simulink library "HEV_Electrical_Lib"  (R2024b)
settings: Solver=ode23t  StartTime=0.0  StopTime=10  MaxStep=1e-3  RelTol=1e-3
values from neighbouring files (symbols this model uses):
  Ts = 2e-6    (= 2e-06)    [param.m]
undefined symbols (not defined in the file or in its folder): DiscIntNeverNeededParam, HEV_Param, magnitude
libraries: fl_lib x73, nesl_utility x30, spsCurrentMeasurementLib x23, spsIdealSwitchLib x12, spsVoltageMeasurementLib x11, simulink_extras x8, spsControlledCurrentSourceLib x7, spsSeriesRLCBranchLib x6, simulink x6, spsControlledVoltageSourceLib x5, spsPermanentMagnetSynchronousMachineLib x4, spsUniversalBridgeLib x3
(part 3 of 4)

== system HEV_Electrical_Lib/Mean Value/Synchronous Motor & Drive/Torque limitation ==
  N rad/s : Inport
  Torque : Inport  Port=2
  Abs1 : Abs
  Gain : Gain  Gain=-1
  Saturation Dynamic : simulink/Discontinuities/Saturation Dynamic  OutMin=[]  OutMax=[]  OutDataTypeStr=Inherit: Same as second input  OutDataType=sfix(16)  OutScaling=2^-10  DoSatur=off
  Torque vs speed profile : Lookup  InputValues=HEV_Param.Motor.TorqSpdLUT.SpeedRPM*pi/30  Table=HEV_Param.Motor.TorqSpdLUT.TorqueNm  SaturateOnIntegerOverflow=off
  torque : Outport  VectorParamsAs1DForOutWhenUnconnected=off
  wires:
  Gain/1 -> Saturation Dynamic/3
  Torque/1 -> Saturation Dynamic/2
  Saturation Dynamic/1 -> torque/1
  Torque vs speed profile/1 -> Gain/1, Saturation Dynamic/1
  Abs1/1 -> Torque vs speed profile/1
  N rad/s/1 -> Abs1/1

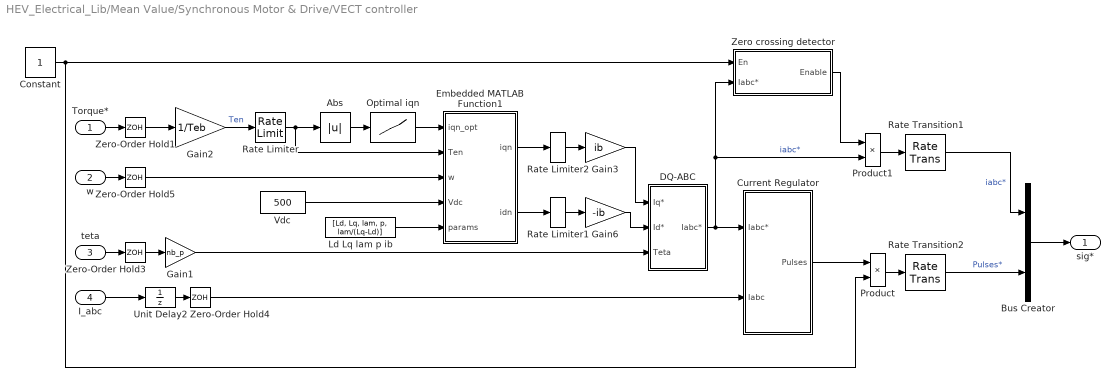
== system HEV_Electrical_Lib/Mean Value/Synchronous Motor & Drive/VECT controller ==
  Torque* : Inport
  w : Inport  Port=2
  teta : Inport  Port=3
  I_abc : Inport  Port=4
  Abs : Abs  SaturateOnIntegerOverflow=off
  Bus Creator : BusCreator  Inputs=2
  Constant : Constant
  Current Regulator : Subsystem
  DQ-ABC : Subsystem
  Embedded MATLAB Function1 : MATLAB Function  TreatAsAtomicUnit=on  SystemSampleTime=Ts_vect
  Gain1 : Gain  Gain=nb_p  SaturateOnIntegerOverflow=on  OutDataTypeStr=Inherit: Same as input  ParamDataTypeStr=Inherit: Same as input
  Gain2 : Gain  Gain=1/Teb  SaturateOnIntegerOverflow=on  OutDataTypeStr=Inherit: Same as input  ParamDataTypeStr=Inherit: Same as input
  Gain3 : Gain  Gain=ib  SaturateOnIntegerOverflow=on  OutDataTypeStr=Inherit: Same as input  ParamDataTypeStr=Inherit: Same as input
  Gain6 : Gain  Gain=-ib  SaturateOnIntegerOverflow=on  OutDataTypeStr=Inherit: Same as input  ParamDataTypeStr=Inherit: Same as input
  Ld Lq lam p ib : Constant  Value=[Ld, Lq, lam, p, lam/(Lq-Ld)]
  Optimal iqn : Lookup  InputValues=ten  Table=iqn  SaturateOnIntegerOverflow=off
  Product : Product  RndMeth=Zero
  Product1 : Product  RndMeth=Zero
  Rate Limiter : RateLimiter  RisingSlewLimit=10  FallingSlewLimit=-10  LinearizeAsGain=off
  Rate Limiter1 : RateLimiter  RisingSlewLimit=100  FallingSlewLimit=-100  SampleTimeMode=inherited
  Rate Limiter2 : RateLimiter  RisingSlewLimit=100  FallingSlewLimit=-100  SampleTimeMode=inherited
  Rate Transition1 : RateTransition
  Rate Transition2 : RateTransition
  Unit Delay2 : UnitDelay  SampleTime=-1  HasFrameUpgradeWarning=on
  Vdc : Constant  Value=500
  Zero crossing detector : Subsystem
  Zero-Order Hold{1,3..5} (4 alike) : ZeroOrderHold  SampleTime=Ts_vect
  sig* : Outport  VectorParamsAs1DForOutWhenUnconnected=off
  wires:
  Rate Limiter/1 -> Embedded MATLAB Function1/2(Ten), Abs/1
  Rate Limiter1/1 -> Gain6/1
  Rate Limiter2/1 -> Gain3/1
  Constant/1 -> Product/2, Zero crossing detector/1(En)
  Zero crossing detector/1(Enable) -> Product1/1
  Product1/1 -> Rate Transition1/1
  Product/1 -> Rate Transition2/1
  Current Regulator/1(Pulses) -> Product/1
  Rate Transition1/1 -> Bus Creator/1  "iabc*"
  Rate Transition2/1 -> Bus Creator/2  "Pulses*"
  Bus Creator/1 -> sig*/1
  Vdc/1 -> Embedded MATLAB Function1/4(Vdc)
  Abs/1 -> Optimal iqn/1
  Optimal iqn/1 -> Embedded MATLAB Function1/1(iqn_opt)
  Embedded MATLAB Function1/1(iqn) -> Rate Limiter2/1
  Ld Lq lam p ib/1 -> Embedded MATLAB Function1/5(params)
  Zero-Order Hold5/1 -> Embedded MATLAB Function1/3(w)
  Gain2/1 -> Rate Limiter/1  "Ten"
  Embedded MATLAB Function1/2(idn) -> Rate Limiter1/1
  w/1 -> Zero-Order Hold5/1
  Zero-Order Hold1/1 -> Gain2/1
  Gain6/1 -> DQ-ABC/2("Id* ")
  Gain3/1 -> DQ-ABC/1("Iq* ")
  Torque*/1 -> Zero-Order Hold1/1
  I_abc/1 -> Unit Delay2/1
  DQ-ABC/1(Iabc*) -> Product1/2, Zero crossing detector/2(Iabc*), Current Regulator/1(Iabc*)  "iabc*"
  Gain1/1 -> DQ-ABC/3(Teta)
  Zero-Order Hold3/1 -> Gain1/1
  teta/1 -> Zero-Order Hold3/1
  Zero-Order Hold4/1 -> Current Regulator/2(Iabc)
  Unit Delay2/1 -> Zero-Order Hold4/1

== system HEV_Electrical_Lib/Subsystem/System Level/Current Sensor SyncMot ==
  Current Sensor : fl_lib/Electrical/Electrical Sensors/Current Sensor
  PS-Simulink Converter : nesl_utility/PS-Simulink Converter  PhysicalDomain=network_engine_domain  SubClassName=ps_output  LeftPortType=input  RightPortType=output  PseudoPeriodic=off  Frequencies=[]  VectorFormat=1-D array  Unit=A  AffineConversion=off
  + : PMIOPort  Side=Left
  - : PMIOPort  Port=2  Side=Right
  tag scope: Mot_Current_SYS=global
  wires:
  PS-Simulink Converter/1 -> [Mot_Current_SYS]
  connections:
  -/RConn1 -- Current Sensor/RConn2
  +/RConn1 -- Current Sensor/LConn1
  Current Sensor/RConn1 -- PS-Simulink Converter/LConn1

== system HEV_Electrical_Lib/Subsystem/System Level/DC-DC Converter ==
  Calcuate Input Current Pout+PLoss = Pin : Subsystem
  Control Bus Voltage : Subsystem
  Controlled Current Source : fl_lib/Electrical/Electrical Sources/Controlled Current Source
  Controlled Voltage Source : fl_lib/Electrical/Electrical Sources/Controlled Voltage Source
  Current Sensor : Subsystem
  Load Dependant Losses : fl_lib/Electrical/Electrical Elements/Resistor  R=RLoadLoss Ohm  i_specify=off  i_priority=High  i=0 A  i_nominal_specify=off  i_nominal_value=1  i_nominal_unit=A  v_specify=off  v_priority=High  v=0 V  v_nominal_specify=off  v_nominal_value=1  v_nominal_unit=V
  PS Constant : fl_lib/Physical Signals/Sources/PS Constant  constant=Vout V
  Subsystem3 : Subsystem
      mask Display: disp('S')
  Thermal Model : Subsystem
  Voltage Sensor : Subsystem
  Voltage Sensor Bus : Subsystem
  " Batt+" : PMIOPort  Tag=PMCPort  Side=Left
  " Batt-" : PMIOPort  Tag=PMCPort  Port=2  Side=Left
  " Bus+" : PMIOPort  Tag=PMCPort  Port=3  Side=Right
  " Bus-" : PMIOPort  Tag=PMCPort  Port=4  Side=Right
  connections:
  Calcuate Input Current Pout+PLoss = Pin/RConn1 -- Subsystem3/RConn1
  Current Sensor/RConn1 -- Calcuate Input Current Pout+PLoss = Pin/LConn2
  Voltage Sensor/RConn1 -- Calcuate Input Current Pout+PLoss = Pin/LConn1
  Voltage Sensor Bus/LConn1 -- Load Dependant Losses/LConn1 -- Current Sensor/RConn2
  Current Sensor/LConn1 -- " Bus+"/RConn1
  Voltage Sensor Bus/RConn1 -- Controlled Voltage Source/RConn2 -- " Bus-"/RConn1
  Load Dependant Losses/RConn1 -- Controlled Voltage Source/LConn1
  Voltage Sensor/RConn2 -- Controlled Current Source/RConn2 -- " Batt-"/RConn1
  Voltage Sensor/LConn1 -- Controlled Current Source/LConn1 -- " Batt+"/RConn1
  Control Bus Voltage/RConn1 -- Controlled Voltage Source/RConn1
  PS Constant/RConn1 -- Control Bus Voltage/LConn2
  Subsystem3/LConn1 -- Controlled Current Source/RConn1
  Voltage Sensor Bus/RConn2 -- Control Bus Voltage/LConn1 -- Calcuate Input Current Pout+PLoss = Pin/LConn3
  Thermal Model/LConn1 -- Calcuate Input Current Pout+PLoss = Pin/RConn2

== system HEV_Electrical_Lib/Subsystem/System Level/Electrical Measurements ==
  Bus Selector : BusSelector  OutputSignals=Voltage (V),Current (A),SOC (%)
  Mux : Mux  Inputs=2
  Mux1 : Mux  Inputs=3
  Mux2 : Mux  Inputs=3
  Mux3 : Mux
  Mux4 : Mux  Inputs=2
  Product1 : Product  RndMeth=Zero
  Product2 : Product  RndMeth=Zero
  Product3 : Product  RndMeth=Zero
  tag scope: Electricals=global, Power=global
  wires:
  Mux4/1 -> Mux3/1
  Mux3/1 -> [Electricals]
  [DC_Bus_SYS] -> Mux4/2, Mux4/1, Mux/1, Product1/2, Product2/2
  Bus Selector/3 -> Mux3/4  "<SOC (%)>"
  [Gen_Current_SYS] -> Mux2/3, Product1/1
  Mux2/1 -> Mux3/3  "Current (Motor, Battery, Generator)"
  Mux/1 -> Mux3/2  "Voltage (DC bus, Battery)"
  Bus Selector/2 -> Mux2/2, Product3/2  "<Current (A)>"
  Bus Selector/1 -> Product3/1, Mux/2  "<Voltage (V)>"
  [Batt_Measures] -> Bus Selector/1
  Mux1/1 -> [Power]
  [Mot_Current_SYS] -> Mux2/1, Product2/1
  Product3/1 -> Mux1/3  "Battery power (W)"
  Product1/1 -> Mux1/2  "Generator power (W)"
  Product2/1 -> Mux1/1  "Motor Power (W)"

== system HEV_Electrical_Lib/Subsystem/System Level/Speed Sensor SyncMot ==
  MRRef : fl_lib/Mechanical/Rotational Elements/Mechanical Rotational Reference
  PS-Simulink Converter : nesl_utility/PS-Simulink Converter  PhysicalDomain=network_engine_domain  SubClassName=ps_output  LeftPortType=input  RightPortType=output  PseudoPeriodic=off  Frequencies=[]  VectorFormat=1-D array  Unit=rpm  AffineConversion=off
  Rotational Motion Sensor : fl_lib/Mechanical/Mechanical Sensors/Ideal Rotational Motion Sensor  reference=foundation.enum.MeasurementReference.difference  acceleration_port=false  velocity_port=true  position_port=true  wrap_angle=simscape.enum.onoff.off  offset=0 rad
  Sh : PMIOPort  Side=Left
  Sh1 : PMIOPort  Port=2  Side=Right
  tag scope: Mot_RPM_SYS=global
  wires:
  PS-Simulink Converter/1 -> [Mot_RPM_SYS]  "Mot_RPM"
  connections:
  Rotational Motion Sensor/RConn1 -- MRRef/LConn1
  Sh1/RConn1 -- Rotational Motion Sensor/LConn1 -- Sh/RConn1
  PS-Simulink Converter/LConn1 -- Rotational Motion Sensor/RConn2

== system HEV_Electrical_Lib/Subsystem/System Level/Synchronous Motor & Drive ==
  TReq : Inport
  GF : Subsystem
      mask Display: disp('GF')
  Inertia : fl_lib/Mechanical/Rotational Elements/Inertia  inertia=HEV_Param.Motor.Shaft_Inertia kg*m^2  num_ports=foundation.enum.numPorts2.one  w_specify=on  w_priority=High  w=0 rad/s  w_nominal_specify=off  w_nominal_value=1  w_nominal_unit=rad/s  t_specify=off  t_priority=High  t=0 N*m  t_nominal_specify=off  t_nominal_value=1  t_nominal_unit=N*m
  MRRef : fl_lib/Mechanical/Rotational Elements/Mechanical Rotational Reference
  Motor & Drive : sdl_lib/Engines & Motors/Motor & Drive  Commented=on  torque_max=10 N*m  power_max=5000 W  Tc=0.01 s  eff=100  w_eff=3750 rpm  T_eff=10 N*m  thermal_port=simscape.enum.thermaleffects.omit  thermal_mass=100 J/K  temperature_specify=off  temperature_priority=High  temperature=300 K  temperature_nominal_specify=off  temperature_nominal_value=1  temperature_nominal_unit=K
      settings: InternalSimscapePortConfiguration="{\"Bottom\":[],\"Left\":[{\"id\":\"Vp\",\"label\":\"+\",\"type\":\"foundation.electrical.electrical\"},{\"id\":\"Tr\",\"label\":\"Tr\",\"type\":\"input\"},{\"id\":\"R\",\"label\":\"R\",\"type\":\"foundation.mechanical.rotational.rotational\"}],\"Right\":[{\"id\":\"Vm\",\"label\":\"-\",\"type\":\"foundation.electrical.electrical\"},{\"id\":\"Omega\",\"label\":\"w\",\"type\":\"output\"},{\"id\":\"C\",\"label\":\"C\",\"type\":\"foundation.mechanical.rotational.rotational\"}],\"Top\":[]}"
  PS Terminator1 : Subsystem
      mask Display:
      | plot([0 0.9],[0.5 0.5]);
      | plot([0.5 0.9],[0.3 0.3]);
      | plot([0.5 0.9],[0.7 0.7]);
      | plot([0.9 0.9],[0.7 0.3]);
  Power Sensor : Subsystem
      mask Display: disp('S')
  Power and Torque Sensor : Subsystem
      mask Display: disp('S')
  Servomotor : ee_lib/Electromechanical/Motor & Drive (System Level)  torque_speed_param=1  overtorque_param=ee.enum.electromech.overtorque.no  T_t=HEV_Param.Motor.TorqSpdLUT.TorqueNm N*m  T_t_intermittent=[.36, .32, .28, 0] N*m  T_t_2D=[.09, .09, .09; .08, .08, .08; .07, .07, .07; 0, 0, 0] N*m  T_t_intermittent_2D=[.36, .36, .36; .32, .32, .32; .28, .28, .28; 0, 0, 0] N*m  w_t=HEV_Param.Motor.TorqSpdLUT.SpeedRPM rpm  vdc_t=[6, 12, 24] V  torque_max=0.1 N*m  power_max=30 W  torque_max_intermittent=0.4 N*m  power_max_intermittent=120 W  time_overtorque=30 s  time_recover=60 s  Tc=HEV_Param.Motor.TorqueControl_TimeConst s  EnableSwitch=simscape.enum.onoff.off  losses_param=1  eff=HEV_Param.Motor.Efficiency  w_eff=2000 rpm  T_eff=200 N*m  Piron=0 W  Pbase=0 W  w_eff_vec=[-8000 -4000 0 4000 8000] rpm  T_eff_vec=[0 0.03 0.06 0.09] N*m  v_eff_vec=[100, 250, 400] V  losses_mat=[1.49 1.67 2.21 3.10; 0.42 0.69 1.14 2.03; 0.06 0.24 0.78 1.68; 0.42 0.69 1.14 2.03; 1.49 1.67 2.21 3.10] W  efficiency_mat=[95 95 95 95; 95 95 95 95; 95 95 95 95; 95 95 95 95; 95 95 95 95]  losses_mat_3D=ones(5, 4, 3) W  efficiency_mat_3D=95 * ones(5, 4, 3)  Res=HEV_Param.Motor.Series_Resistance Ohm  J=0 kg*m^2  lam=HEV_Param.Motor.Damping N*m/(rad/s)  speed0=0 rpm  fault_condition=1  fault_threshold=0.5  faulted_specify=off  faulted_priority=None  faulted=0  faulted_nominal_specify=off  faulted_nominal_value=1  faulted_nominal_unit=1  isSwitchedOff_specify=off  isSwitchedOff_priority=None  isSwitchedOff=0  isSwitchedOff_nominal_specify=off  isSwitchedOff_nominal_value=1  isSwitchedOff_nominal_unit=1  torqueLimitContinuous_specify=off  torqueLimitContinuous_priority=None  torqueLimitContinuous=0 N*m  torqueLimitContinuous_nominal_specify=off  torqueLimitContinuous_nominal_value=1  torqueLimitContinuous_nominal_unit=N*m  alpha=3.93e-3 1/K  Tmeas=25 degC  Tmeas2=125 degC  losses_mat_T2=[1.49, 1.74, 2.49, 3.74; .42, .67, 1.42, 2.67; .06, .31, 1.06, 2.31; .42, .67, 1.42, 2.67; 1.49, 1.74, 2.49, 3.74] W  efficiency_mat_T2=[95, 95, 95, 95; 95, 95, 95, 95; 95, 95, 95, 95; 95, 95, 95, 95; 95, 95, 95, 95]  losses_mat_3D_T2=ones(5, 4, 3) W  efficiency_mat_3D_T2=95 * ones(5, 4, 3)  thermal_mass=100 J/K  initial_temperature=25 degC
  Vcc : PMIOPort  Side=Right
  Gnd : PMIOPort  Port=2  Side=Right
  Shaft : PMIOPort  Port=3  Side=Right
  wires:
  TReq/1 -> GF/1(In1)
  connections:
  Servomotor/RConn3 -- MRRef/LConn1
  Servomotor/LConn3 -- Power and Torque Sensor/LConn1
  Servomotor/LConn2 -- GF/RConn1
  Servomotor/LConn1 -- Power Sensor/RConn1
  Vcc/RConn1 -- Power Sensor/LConn1
  Gnd/RConn1 -- Servomotor/RConn1 -- Power Sensor/LConn2
  Servomotor/RConn2 -- PS Terminator1/LConn1
  Inertia/LConn1 -- Power and Torque Sensor/RConn1 -- Shaft/RConn1

== system HEV_Electrical_Lib/Subsystem/System Level/Voltage Sensor ==
  PS-Simulink Converter : nesl_utility/PS-Simulink Converter  PhysicalDomain=network_engine_domain  SubClassName=ps_output  LeftPortType=input  RightPortType=output  PseudoPeriodic=off  Frequencies=[]  VectorFormat=1-D array  Unit=V  AffineConversion=off
  Voltage Sensor : fl_lib/Electrical/Electrical Sensors/Voltage Sensor
  + : PMIOPort  Side=Left
  - : PMIOPort  Port=2  Side=Right
  tag scope: DC_Bus_SYS=global
  wires:
  PS-Simulink Converter/1 -> [DC_Bus_SYS]
  connections:
  -/RConn1 -- Voltage Sensor/RConn2
  +/RConn1 -- Voltage Sensor/LConn1
  Voltage Sensor/RConn1 -- PS-Simulink Converter/LConn1

== system HEV_Electrical_Lib/Detailed/DC//DC Converter/PWM/Sawtooth generator ==
  1\ib3 : Gain  Gain=2  SaturateOnIntegerOverflow=on  OutDataTypeStr=Inherit: Same as input  ParamDataTypeStr=Inherit: Same as input
  Constant1 : Constant  Value=20000
  Constant2 : Constant  Value=2
  Constant3 : Constant
  Discrete-Time Integrator : DiscreteIntegrator  IntegratorMethod=Integration: Trapezoidal  ExternalReset=rising  SampleTime=Ts  UpperSaturationLimit=1.5  LowerSaturationLimit=-1.5  ICPrevOutput=DiscIntNeverNeededParam  ICPrevScaledInput=DiscIntNeverNeededParam
  Relational Operator1 : RelationalOperator  InputSameDT=off
  Sum1 : Sum  Inputs=+-  InputSameDT=on  SaturateOnIntegerOverflow=on  OutDataTypeStr=Inherit: Same as first input
  Unit Delay : UnitDelay  SampleTime=Ts  HasFrameUpgradeWarning=on
  Out : Outport  VectorParamsAs1DForOutWhenUnconnected=off
  wires:
  Constant1/1 -> 1\ib3/1
  Discrete-Time Integrator/1 -> Relational Operator1/1, Sum1/1
  Constant2/1 -> Relational Operator1/2
  Relational Operator1/1 -> Unit Delay/1
  Unit Delay/1 -> Discrete-Time Integrator/2
  Sum1/1 -> Out/1
  Constant3/1 -> Sum1/2
  1\ib3/1 -> Discrete-Time Integrator/1

== system HEV_Electrical_Lib/Detailed/DC//DC Converter/PWM/Thermal Model ==
  IBus : Inport
  1/Mc : Gain  Gain=1/(HEV_Param.DCDCConv.Thermal_Mass*HEV_Param.DCDCConv.Specific_Heat)  SaturateOnIntegerOverflow=on  OutDataTypeStr=Inherit: Same as input  ParamDataTypeStr=Inherit: Same as input
  Air_Temp : Constant  Value=HEV_Param.DCDCConv.Air_Temperature-273
  Heat Losses : Gain  Gain=HEV_Param.DCDCConv.Convection.Area/HEV_Param.DCDCConv.Convection.HT_Coefficient  SaturateOnIntegerOverflow=on  OutDataTypeStr=Inherit: Same as input  ParamDataTypeStr=Inherit: Same as input
  Integrator : Integrator  InitialCondition=HEV_Param.DCDCConv.Initial_Temperature
  Subsystem : Subsystem
  Sum1 : Sum  Inputs=|+-  InputSameDT=on  SaturateOnIntegerOverflow=on  OutDataTypeStr=Inherit: Same as first input
  Sum2 : Sum  Inputs=|+-  InputSameDT=on  SaturateOnIntegerOverflow=on  OutDataTypeStr=Inherit: Same as first input
  tag scope: DCDC_SYS=global
  wires:
  Sum1/1 -> 1/Mc/1
  Sum2/1 -> Heat Losses/1
  Heat Losses/1 -> Sum1/2
  1/Mc/1 -> Integrator/1
  Integrator/1 -> [DCDC_SYS], Sum2/1  "DCDC_Temp"
  IBus/1 -> Subsystem/1(IBus)
  Subsystem/1(Heat Flow) -> Sum1/1  "Heat In"
  Air_Temp/1 -> Sum2/2

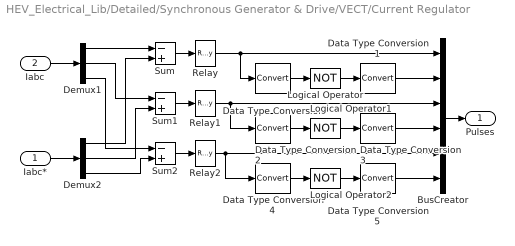
== system HEV_Electrical_Lib/Detailed/Synchronous Generator & Drive/VECT/Current Regulator ==
  Iabc* : Inport
  Iabc : Inport  Port=2
  BusCreator : BusCreator  Inputs=6
  Data Type Conversion{,1..5} (6 alike) : DataTypeConversion
  Demux1 : Demux  Outputs=3
      settings: DisplayOption=none
  Demux2 : Demux  Outputs=3
      settings: DisplayOption=none
  Logical Operator : Logic  Operator=NOT
  Logical Operator1 : Logic  Operator=NOT
  Logical Operator2 : Logic  Operator=NOT
  Relay : Relay  OnSwitchValue=h/2  OffSwitchValue=-h/2
  Relay1 : Relay  OnSwitchValue=h/2  OffSwitchValue=-h/2
  Relay2 : Relay  OnSwitchValue=h/2  OffSwitchValue=-h/2
  Sum : Sum  Inputs=-+  InputSameDT=on  SaturateOnIntegerOverflow=on  OutDataTypeStr=Inherit: Same as first input
  Sum1 : Sum  Inputs=-+  InputSameDT=on  SaturateOnIntegerOverflow=on  OutDataTypeStr=Inherit: Same as first input
  Sum2 : Sum  Inputs=-+  InputSameDT=on  SaturateOnIntegerOverflow=on  OutDataTypeStr=Inherit: Same as first input
  Pulses : Outport  InitialOutput=0  VectorParamsAs1DForOutWhenUnconnected=off
  wires:
  Logical Operator2/1 -> Data Type Conversion5/1
  Logical Operator1/1 -> Data Type Conversion3/1
  Logical Operator/1 -> Data Type Conversion1/1
  Relay2/1 -> BusCreator/5, Data Type Conversion4/1
  Relay1/1 -> BusCreator/3, Data Type Conversion2/1
  Relay/1 -> BusCreator/1, Data Type Conversion/1
  Iabc*/1 -> Demux2/1
  Demux2/1 -> Sum/2
  Demux2/2 -> Sum1/2
  Demux2/3 -> Sum2/2
  Demux1/3 -> Sum2/1
  Sum2/1 -> Relay2/1
  Iabc/1 -> Demux1/1
  BusCreator/1 -> Pulses/1
  Demux1/2 -> Sum1/1
  Demux1/1 -> Sum/1
  Sum1/1 -> Relay1/1
  Sum/1 -> Relay/1
  Data Type Conversion/1 -> Logical Operator/1
  Data Type Conversion1/1 -> BusCreator/2
  Data Type Conversion2/1 -> Logical Operator1/1
  Data Type Conversion3/1 -> BusCreator/4
  Data Type Conversion4/1 -> Logical Operator2/1
  Data Type Conversion5/1 -> BusCreator/6

== system HEV_Electrical_Lib/Detailed/Synchronous Generator & Drive/VECT/DQ-ABC ==
  "Iq* " : Inport
  "Id* " : Inport  Port=2
  Teta : Inport  Port=3
  Fcn : Fcn  Expr=sin(u)
  Fcn1 : Fcn  Expr=cos(u)
  Gain2 : Gain  SaturateOnIntegerOverflow=on  OutDataTypeStr=Inherit: Same as input  ParamDataTypeStr=Inherit: Same as input
  Gain3 : Gain  SaturateOnIntegerOverflow=on  OutDataTypeStr=Inherit: Same as input  ParamDataTypeStr=Inherit: Same as input
  Gain4 : Gain  SaturateOnIntegerOverflow=on  OutDataTypeStr=Inherit: Same as input  ParamDataTypeStr=Inherit: Same as input
  Mux : Mux
  Mux2 : Mux  Inputs=3
  ia : Fcn  Expr=-u[3]*u[2] + u[4]*u[1]
  ib : Fcn  Expr=(-u[1]+1.7320508*u[2])*u[4]*0.5+(u[2]+1.7320508*u[1])*u[3]*0.5
  ic : Sum  Inputs=--  InputSameDT=on  SaturateOnIntegerOverflow=on  OutDataTypeStr=Inherit: Same as first input
  Iabc* : Outport  InitialOutput=0  VectorParamsAs1DForOutWhenUnconnected=off
  wires:
  ib/1 -> ic/1, Gain3/1
  ia/1 -> ic/2, Gain2/1
  Gain2/1 -> Mux2/1
  Gain4/1 -> Mux2/3
  ic/1 -> Gain4/1
  Gain3/1 -> Mux2/2
  "Iq* "/1 -> Mux/4
  "Id* "/1 -> Mux/3
  Teta/1 -> Fcn/1, Fcn1/1
  Mux/1 -> ia/1, ib/1
  Mux2/1 -> Iabc*/1
  Fcn1/1 -> Mux/1
  Fcn/1 -> Mux/2

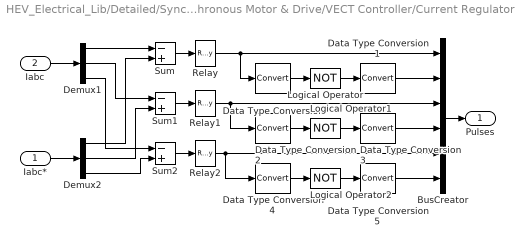
== system HEV_Electrical_Lib/Detailed/Synchronous Motor & Drive/VECT Controller/Current Regulator1 ==
  Iabc* : Inport
  Iabc : Inport  Port=2
  BusCreator : BusCreator  Inputs=6
  Data Type Conversion{,1..5} (6 alike) : DataTypeConversion
  Demux1 : Demux  Outputs=3
      settings: DisplayOption=none
  Demux2 : Demux  Outputs=3
      settings: DisplayOption=none
  Logical Operator : Logic  Operator=NOT
  Logical Operator1 : Logic  Operator=NOT
  Logical Operator2 : Logic  Operator=NOT
  Relay : Relay  OnSwitchValue=h/2  OffSwitchValue=-h/2
  Relay1 : Relay  OnSwitchValue=h/2  OffSwitchValue=-h/2
  Relay2 : Relay  OnSwitchValue=h/2  OffSwitchValue=-h/2
  Sum : Sum  Inputs=-+  InputSameDT=on  SaturateOnIntegerOverflow=on  OutDataTypeStr=Inherit: Same as first input
  Sum1 : Sum  Inputs=-+  InputSameDT=on  SaturateOnIntegerOverflow=on  OutDataTypeStr=Inherit: Same as first input
  Sum2 : Sum  Inputs=-+  InputSameDT=on  SaturateOnIntegerOverflow=on  OutDataTypeStr=Inherit: Same as first input
  Pulses : Outport  InitialOutput=0  VectorParamsAs1DForOutWhenUnconnected=off
  wires:
  Data Type Conversion5/1 -> BusCreator/6
  Data Type Conversion4/1 -> Logical Operator2/1
  Data Type Conversion3/1 -> BusCreator/4
  Data Type Conversion2/1 -> Logical Operator1/1
  Data Type Conversion1/1 -> BusCreator/2
  Data Type Conversion/1 -> Logical Operator/1
  Sum/1 -> Relay/1
  Sum1/1 -> Relay1/1
  Demux1/1 -> Sum/1
  Demux1/2 -> Sum1/1
  BusCreator/1 -> Pulses/1
  Iabc/1 -> Demux1/1
  Sum2/1 -> Relay2/1
  Demux1/3 -> Sum2/1
  Demux2/3 -> Sum2/2
  Demux2/2 -> Sum1/2
  Demux2/1 -> Sum/2
  Iabc*/1 -> Demux2/1
  Relay/1 -> Data Type Conversion/1, BusCreator/1
  Relay1/1 -> Data Type Conversion2/1, BusCreator/3
  Relay2/1 -> Data Type Conversion4/1, BusCreator/5
  Logical Operator/1 -> Data Type Conversion1/1
  Logical Operator1/1 -> Data Type Conversion3/1
  Logical Operator2/1 -> Data Type Conversion5/1

== system HEV_Electrical_Lib/Detailed/Synchronous Motor & Drive/VECT Controller/DQ-ABC ==
  "Iq* " : Inport
  "Id* " : Inport  Port=2
  Teta : Inport  Port=3
  Fcn : Fcn  Expr=sin(u)
  Fcn1 : Fcn  Expr=cos(u)
  Gain2 : Gain  SaturateOnIntegerOverflow=on  OutDataTypeStr=Inherit: Same as input  ParamDataTypeStr=Inherit: Same as input
  Gain3 : Gain  SaturateOnIntegerOverflow=on  OutDataTypeStr=Inherit: Same as input  ParamDataTypeStr=Inherit: Same as input
  Gain4 : Gain  SaturateOnIntegerOverflow=on  OutDataTypeStr=Inherit: Same as input  ParamDataTypeStr=Inherit: Same as input
  Mux : Mux
  Mux2 : Mux  Inputs=3
  ia : Fcn  Expr=-u[3]*u[2] + u[4]*u[1]
  ib : Fcn  Expr=(-u[1]+1.7320508*u[2])*u[4]*0.5+(u[2]+1.7320508*u[1])*u[3]*0.5
  ic : Sum  Inputs=--  InputSameDT=on  SaturateOnIntegerOverflow=on  OutDataTypeStr=Inherit: Same as first input
  Iabc* : Outport  InitialOutput=0  VectorParamsAs1DForOutWhenUnconnected=off
  wires:
  ib/1 -> ic/1, Gain3/1
  ia/1 -> ic/2, Gain2/1
  Gain2/1 -> Mux2/1
  Gain4/1 -> Mux2/3
  ic/1 -> Gain4/1
  Gain3/1 -> Mux2/2
  "Iq* "/1 -> Mux/4
  "Id* "/1 -> Mux/3
  Teta/1 -> Fcn/1, Fcn1/1
  Mux/1 -> ia/1, ib/1
  Mux2/1 -> Iabc*/1
  Fcn1/1 -> Mux/1
  Fcn/1 -> Mux/2

== system HEV_Electrical_Lib/Mean Value/DC//DC Converter/Boost Converter Average-Values/Thermal Model ==
  IBus : Inport
  1/Mc : Gain  Gain=1/(HEV_Param.DCDCConv.Thermal_Mass*HEV_Param.DCDCConv.Specific_Heat)  SaturateOnIntegerOverflow=on  OutDataTypeStr=Inherit: Same as input  ParamDataTypeStr=Inherit: Same as input
  Air_Temp : Constant  Value=HEV_Param.DCDCConv.Air_Temperature-273
  Heat Losses : Gain  Gain=HEV_Param.DCDCConv.Convection.Area/HEV_Param.DCDCConv.Convection.HT_Coefficient  SaturateOnIntegerOverflow=on  OutDataTypeStr=Inherit: Same as input  ParamDataTypeStr=Inherit: Same as input
  Integrator : Integrator  InitialCondition=HEV_Param.DCDCConv.Initial_Temperature
  Subsystem : Subsystem
  Sum1 : Sum  Inputs=|+-  InputSameDT=on  SaturateOnIntegerOverflow=on  OutDataTypeStr=Inherit: Same as first input
  Sum2 : Sum  Inputs=|+-  InputSameDT=on  SaturateOnIntegerOverflow=on  OutDataTypeStr=Inherit: Same as first input
  tag scope: DCDC_SYS=global
  wires:
  Air_Temp/1 -> Sum2/2
  Subsystem/1(Heat Flow) -> Sum1/1  "Heat In"
  IBus/1 -> Subsystem/1(IBus)
  Integrator/1 -> Sum2/1, [DCDC_SYS]  "DCDC_Temp"
  1/Mc/1 -> Integrator/1
  Heat Losses/1 -> Sum1/2
  Sum2/1 -> Heat Losses/1
  Sum1/1 -> 1/Mc/1

== system HEV_Electrical_Lib/Mean Value/Synchronous Generator & Drive/Three-phase Inverter/Activation Switches ==
  gate : Inport
  Ideal Switch1 : spsIdealSwitchLib/Ideal Switch  Ron=2*Ron  Lon=0  IC=1  Rs=1e6  Cs=inf  Measurements=off
  Ideal Switch2 : spsIdealSwitchLib/Ideal Switch  Ron=2*Ron  Lon=0  IC=1  Rs=1e6  Cs=inf  Measurements=off
  Ideal Switch3 : spsIdealSwitchLib/Ideal Switch  Ron=2*Ron  Lon=0  IC=1  Rs=1e6  Cs=inf  Measurements=off
  Ideal Switch4 : spsIdealSwitchLib/Ideal Switch  Ron=2*Ron  Lon=0  IC=0  Rs=1e6  Cs=inf  Measurements=off
  Ideal Switch5 : spsIdealSwitchLib/Ideal Switch  Ron=2*Ron  Lon=0  IC=0  Rs=1e6  Cs=inf  Measurements=off
  Ideal Switch6 : spsIdealSwitchLib/Ideal Switch  Ron=2*Ron  Lon=0  IC=0  Rs=1e6  Cs=inf  Measurements=off
  Logical Operator : Logic  Operator=NOT  AllPortsSameDT=off  OutDataTypeStr=boolean
  A1 : PMIOPort  Side=Left
  a : PMIOPort  Port=2  Side=Right
  B1 : PMIOPort  Port=3  Side=Left
  b : PMIOPort  Port=4  Side=Right
  C1 : PMIOPort  Port=5  Side=Left
  c : PMIOPort  Port=6  Side=Right
  A2 : PMIOPort  Port=7  Side=Left
  B2 : PMIOPort  Port=8  Side=Left
  C2 : PMIOPort  Port=9  Side=Left
  wires:
  gate/1 -> Ideal Switch1/1, Ideal Switch2/1, Ideal Switch3/1, Logical Operator/1
  Logical Operator/1 -> Ideal Switch4/1, Ideal Switch5/1, Ideal Switch6/1
  connections:
  A1/RConn1 -- Ideal Switch1/LConn1
  Ideal Switch1/RConn1 -- a/RConn1 -- Ideal Switch4/RConn1
  B1/RConn1 -- Ideal Switch2/LConn1
  Ideal Switch2/RConn1 -- Ideal Switch5/RConn1 -- b/RConn1
  C1/RConn1 -- Ideal Switch3/LConn1
  Ideal Switch3/RConn1 -- Ideal Switch6/RConn1 -- c/RConn1
  A2/RConn1 -- Ideal Switch4/LConn1
  B2/RConn1 -- Ideal Switch5/LConn1
  C2/RConn1 -- Ideal Switch6/LConn1

== system HEV_Electrical_Lib/Mean Value/Synchronous Generator & Drive/Three-phase Inverter/Id computation ==
  m : Inport
  Vdc : Inport  Port=2
  Demux : Subsystem
  Demux1 : Subsystem
  Gain : Gain  Gain=Ron
  Math Function : Math  Operator=magnitude^2  SignedPower=on
  Math Function1 : Math  Operator=magnitude^2  SignedPower=on
  Math Function2 : Math  Operator=magnitude^2  SignedPower=on
  Product1 : Product  Inputs=*/  SaturateOnIntegerOverflow=on  OutDataTypeStr=Inherit: Same as first input
  Sum1 : Sum  Inputs=+++  SaturateOnIntegerOverflow=on
  Sum2 : Sum  Inputs=|++  SaturateOnIntegerOverflow=on
  Sum3 : Sum  SaturateOnIntegerOverflow=on
  Unit Delay1 : UnitDelay  SampleTime=Ts  HasFrameUpgradeWarning=on
  Unit Delay4 : UnitDelay  InitialCondition=1  SampleTime=Ts  HasFrameUpgradeWarning=on
  Vac x Ia : Product  SaturateOnIntegerOverflow=on  OutDataTypeStr=Inherit: Same as first input
  Vbc x Ib : Product  SaturateOnIntegerOverflow=on  OutDataTypeStr=Inherit: Same as first input
  Zero avoider : Saturate  UpperLimit=inf  LowerLimit=1
  Id : Outport  VectorParamsAs1DForOutWhenUnconnected=off
  wires:
  Sum2/1 -> Unit Delay1/1
  Sum3/1 -> Sum2/1
  Sum1/1 -> Gain/1
  Math Function2/1 -> Sum1/3
  Math Function/1 -> Sum1/1
  Math Function1/1 -> Sum1/2
  Demux1/3(Ic) -> Math Function2/1
  Demux1/2(Ib) -> Math Function1/1
  Demux1/1(Ia) -> Math Function/1
  Unit Delay4/1 -> Zero avoider/1
  Unit Delay1/1 -> Product1/1
  m/1 -> Demux1/1(m), Demux/1(m)
  Vac x Ia/1 -> Sum3/1
  Vbc x Ib/1 -> Sum3/2
  Vdc/1 -> Unit Delay4/1
  Demux/1(Vac) -> Vac x Ia/1
  Demux/2(Ia) -> Vac x Ia/2
  Demux/4(Ib) -> Vbc x Ib/2
  Demux/3(Vbc) -> Vbc x Ib/1
  Gain/1 -> Sum2/2
  Product1/1 -> Id/1
  Zero avoider/1 -> Product1/2

== system HEV_Electrical_Lib/Mean Value/Synchronous Generator & Drive/Three-phase Inverter/Limit detection ==
  note: Limit = 1 saturation mode (voltage mode)
      | Limit = 0 normal mode (current mode)
  note: Low pass filter
  note: Low pass filter
  Vcc : Inport
  ctrl : Inport  Port=2
  Bus Selector1 : BusSelector  OutputSignals=m.Stator current is_d (A),m.Stator current is_q (A),m.Rotor speed wm (rad/s)  OutputAsBus=on
  Discrete Transfer Fcn1 : DiscreteTransferFcn  Numerator=[1-exp(-Ts*Fcs*2*pi)]  Denominator=[1 -exp(-Ts*Fcs*2*pi)]  SampleTime=Ts
  Discrete Transfer Fcn3 : DiscreteTransferFcn  Numerator=[1-exp(-Ts*Fcs*2*pi)]  Denominator=[1 -exp(-Ts*Fcs*2*pi)]  SampleTime=Ts
  Gain1 : Gain  Gain=0.9  SaturateOnIntegerOverflow=on  OutDataTypeStr=Inherit: Same as input  ParamDataTypeStr=Inherit: Same as input
  "Internal Vcc " : Fcn  Expr=pi/2*sqrt((Resistance*u(1)-Lq*p*u(3)*u(2))^2+(Resistance*u(2)+Ld*p*u(3)*u(1)+Flux*p*u(3))^2)
  Relational Operator : RelationalOperator  Operator=>  OutDataTypeStr=boolean  InputSameDT=off
  Relational Operator2 : RelationalOperator  Operator=<  OutDataTypeStr=boolean  InputSameDT=off
  S-R Flip-Flop : simulink_extras/Flip Flops/S-R Flip-Flop  initial_condition=0
  Terminator : Terminator
  Limit : Outport  VectorParamsAs1DForOutWhenUnconnected=off
  wires:
  Vcc/1 -> Discrete Transfer Fcn3/1
  Relational Operator/1 -> S-R Flip-Flop/1
  Relational Operator2/1 -> S-R Flip-Flop/2
  S-R Flip-Flop/1 -> Limit/1
  ctrl/1 -> Bus Selector1/1
  Bus Selector1/1 -> "Internal Vcc "/1
  "Internal Vcc "/1 -> Discrete Transfer Fcn1/1
  Discrete Transfer Fcn1/1 -> Relational Operator/1, Relational Operator2/1
  Gain1/1 -> Relational Operator2/2
  Discrete Transfer Fcn3/1 -> Gain1/1, Relational Operator/2
  S-R Flip-Flop/2 -> Terminator/1

== system HEV_Electrical_Lib/Mean Value/Synchronous Generator & Drive/Three-phase Inverter/Output Resistance correction ==
  note: Vabc
  ctrl : Inport
  1/R : Gain  Gain=1/(100*Resistance)  SaturateOnIntegerOverflow=on  OutDataTypeStr=Inherit: Same as input  ParamDataTypeStr=Inherit: Same as input
  Bus Selector1 : BusSelector  OutputSignals=m.Stator voltage Vs_d (V),m.Stator voltage Vs_q (V),m.Rotor angle thetam (rad)
  Constant : Constant  Value=0
  Discrete Transfer Fcn1 : DiscreteTransferFcn  Numerator=[1-exp(-Ts/.001)]  Denominator=[1 -exp(-Ts/.001)]  SampleTime=Ts
  Discrete Transfer Fcn2 : DiscreteTransferFcn  Numerator=[1-exp(-Ts/.001)]  Denominator=[1 -exp(-Ts/.001)]  SampleTime=Ts
  Fcn : Fcn  Expr=sin(u)
  Fcn1 : Fcn  Expr=cos(u)
  Mux4 : Mux  Inputs=3
  Mux5 : Mux  Inputs=2
  dq0_to_abc Transformation : powerlib_extras/Measurements/dq0_to_abc Transformation
  poles : Gain  Gain=p  SaturateOnIntegerOverflow=on  OutDataTypeStr=Inherit: Same as input  ParamDataTypeStr=Inherit: Same as input
  "Iabc_r " : Outport  VectorParamsAs1DForOutWhenUnconnected=off
  wires:
  1/R/1 -> "Iabc_r "/1
  Bus Selector1/2 -> Discrete Transfer Fcn2/1  "<Stator voltage Vs_q (V)>"
  Bus Selector1/1 -> Discrete Transfer Fcn1/1  "<Stator voltage Vs_d (V)>"
  ctrl/1 -> Bus Selector1/1
  Mux4/1 -> dq0_to_abc Transformation/1
  Fcn/1 -> Mux5/1
  Fcn1/1 -> Mux5/2
  Mux5/1 -> dq0_to_abc Transformation/2
  Constant/1 -> Mux4/3
  dq0_to_abc Transformation/1 -> 1/R/1
  Discrete Transfer Fcn2/1 -> Mux4/2
  Discrete Transfer Fcn1/1 -> Mux4/1
  Bus Selector1/3 -> poles/1  "<Rotor angle thetam (rad)>"
  poles/1 -> Fcn1/1, Fcn/1

== system HEV_Electrical_Lib/Mean Value/Synchronous Generator & Drive/VECT/Current Regulator ==
  Iabc* : Inport
  Iabc : Inport  Port=2
  Demux1 : Demux  Outputs=3
      settings: DisplayOption=none
  Demux2 : Demux  Outputs=3
      settings: DisplayOption=none
  Mux1 : Mux  Inputs=2
  Relay : Relay  OnSwitchValue=0  OffSwitchValue=0
  Relay1 : Relay  OnSwitchValue=0  OffSwitchValue=0
  Relay2 : Relay  OnSwitchValue=0  OffSwitchValue=0
  Sum : Sum  Inputs=-+  InputSameDT=on  SaturateOnIntegerOverflow=on  OutDataTypeStr=Inherit: Same as first input
  Sum1 : Sum  Inputs=-+  InputSameDT=on  SaturateOnIntegerOverflow=on  OutDataTypeStr=Inherit: Same as first input
  Sum2 : Sum  Inputs=-+  InputSameDT=on  SaturateOnIntegerOverflow=on  OutDataTypeStr=Inherit: Same as first input
  Sum3 : Sum  Inputs=+-
  Sum4 : Sum  Inputs=+-
  Pulses : Outport  InitialOutput=0  VectorParamsAs1DForOutWhenUnconnected=off
  wires:
  Sum/1 -> Relay/1
  Sum1/1 -> Relay1/1
  Demux1/1 -> Sum/1
  Demux1/2 -> Sum1/1
  Mux1/1 -> Pulses/1
  Iabc/1 -> Demux1/1
  Sum2/1 -> Relay2/1
  Demux1/3 -> Sum2/1
  Demux2/3 -> Sum2/2
  Demux2/2 -> Sum1/2
  Demux2/1 -> Sum/2
  Iabc*/1 -> Demux2/1
  Relay/1 -> Sum3/1
  Relay1/1 -> Sum3/2, Sum4/1
  Relay2/1 -> Sum4/2
  Sum3/1 -> Mux1/1
  Sum4/1 -> Mux1/2

== system HEV_Electrical_Lib/Mean Value/Synchronous Generator & Drive/VECT/DQ-ABC ==
  "Iq* " : Inport
  "Id* " : Inport  Port=2
  Teta : Inport  Port=3
  Fcn : Fcn  Expr=sin(u)
  Fcn1 : Fcn  Expr=cos(u)
  Gain2 : Gain  SaturateOnIntegerOverflow=on  OutDataTypeStr=Inherit: Same as input  ParamDataTypeStr=Inherit: Same as input
  Gain3 : Gain  SaturateOnIntegerOverflow=on  OutDataTypeStr=Inherit: Same as input  ParamDataTypeStr=Inherit: Same as input
  Gain4 : Gain  SaturateOnIntegerOverflow=on  OutDataTypeStr=Inherit: Same as input  ParamDataTypeStr=Inherit: Same as input
  Mux : Mux
  Mux2 : Mux  Inputs=3
  ia : Fcn  Expr=-u[3]*u[2] + u[4]*u[1]
  ib : Fcn  Expr=(-u[1]+1.7320508*u[2])*u[4]*0.5+(u[2]+1.7320508*u[1])*u[3]*0.5
  ic : Sum  Inputs=--  InputSameDT=on  SaturateOnIntegerOverflow=on  OutDataTypeStr=Inherit: Same as first input
  Iabc* : Outport  InitialOutput=0  VectorParamsAs1DForOutWhenUnconnected=off
  wires:
  ib/1 -> ic/1, Gain3/1
  ia/1 -> ic/2, Gain2/1
  Gain2/1 -> Mux2/1
  Gain4/1 -> Mux2/3
  ic/1 -> Gain4/1
  Gain3/1 -> Mux2/2
  "Iq* "/1 -> Mux/4
  "Id* "/1 -> Mux/3
  Teta/1 -> Fcn/1, Fcn1/1
  Mux/1 -> ia/1, ib/1
  Mux2/1 -> Iabc*/1
  Fcn1/1 -> Mux/1
  Fcn/1 -> Mux/2

== system HEV_Electrical_Lib/Mean Value/Synchronous Generator & Drive/VECT/Zero crossing detector ==
  Iabc* : Inport
  En : Inport  Port=2
  D Latch : simulink_extras/Flip Flops/D Latch
  D Latch1 : simulink_extras/Flip Flops/D Latch
  D Latch2 : simulink_extras/Flip Flops/D Latch
  Data Type Conversion : DataTypeConversion  SaturateOnIntegerOverflow=off  RndMeth=Floor
  Data Type Conversion2 : DataTypeConversion  SaturateOnIntegerOverflow=off  RndMeth=Floor
  Demux : Demux  Outputs=3
  Hit Crossing : HitCross
  Mux : Mux  Inputs=3
  Terminator : Terminator
  Terminator1 : Terminator
  Terminator2 : Terminator
  Enable : Outport  VectorParamsAs1DForOutWhenUnconnected=off
  wires:
  Data Type Conversion/1 -> D Latch/1, D Latch1/1, D Latch2/1
  Hit Crossing/1 -> Demux/1
  Demux/2 -> D Latch1/2
  Demux/3 -> D Latch2/2
  D Latch/1 -> Mux/1
  D Latch1/1 -> Mux/2
  D Latch2/1 -> Mux/3
  Mux/1 -> Data Type Conversion2/1
  Demux/1 -> D Latch/2
  En/1 -> Data Type Conversion/1
  Iabc*/1 -> Hit Crossing/1
  Data Type Conversion2/1 -> Enable/1
  D Latch/2 -> Terminator/1
  D Latch1/2 -> Terminator1/1
  D Latch2/2 -> Terminator2/1

== system HEV_Electrical_Lib/Mean Value/Synchronous Motor & Drive/Three-phase Inverter/Activation Switches ==
  gate : Inport
  Ideal Switch1 : spsIdealSwitchLib/Ideal Switch  Ron=2*Ron  Lon=0  IC=1  Rs=1e6  Cs=inf  Measurements=off
  Ideal Switch2 : spsIdealSwitchLib/Ideal Switch  Ron=2*Ron  Lon=0  IC=1  Rs=1e6  Cs=inf  Measurements=off
  Ideal Switch3 : spsIdealSwitchLib/Ideal Switch  Ron=2*Ron  Lon=0  IC=1  Rs=1e6  Cs=inf  Measurements=off
  Ideal Switch4 : spsIdealSwitchLib/Ideal Switch  Ron=2*Ron  Lon=0  IC=0  Rs=1e6  Cs=inf  Measurements=off
  Ideal Switch5 : spsIdealSwitchLib/Ideal Switch  Ron=2*Ron  Lon=0  IC=0  Rs=1e6  Cs=inf  Measurements=off
  Ideal Switch6 : spsIdealSwitchLib/Ideal Switch  Ron=2*Ron  Lon=0  IC=0  Rs=1e6  Cs=inf  Measurements=off
  Logical Operator : Logic  Operator=NOT  AllPortsSameDT=off  OutDataTypeStr=boolean
  A1 : PMIOPort  Side=Left
  a : PMIOPort  Port=2  Side=Right
  B1 : PMIOPort  Port=3  Side=Left
  b : PMIOPort  Port=4  Side=Right
  C1 : PMIOPort  Port=5  Side=Left
  c : PMIOPort  Port=6  Side=Right
  A2 : PMIOPort  Port=7  Side=Left
  B2 : PMIOPort  Port=8  Side=Left
  C2 : PMIOPort  Port=9  Side=Left
  wires:
  Logical Operator/1 -> Ideal Switch6/1, Ideal Switch5/1, Ideal Switch4/1
  gate/1 -> Logical Operator/1, Ideal Switch3/1, Ideal Switch2/1, Ideal Switch1/1
  connections:
  C2/RConn1 -- Ideal Switch6/LConn1
  B2/RConn1 -- Ideal Switch5/LConn1
  A2/RConn1 -- Ideal Switch4/LConn1
  c/RConn1 -- Ideal Switch6/RConn1 -- Ideal Switch3/RConn1
  C1/RConn1 -- Ideal Switch3/LConn1
  b/RConn1 -- Ideal Switch5/RConn1 -- Ideal Switch2/RConn1
  B1/RConn1 -- Ideal Switch2/LConn1
  Ideal Switch4/RConn1 -- a/RConn1 -- Ideal Switch1/RConn1
  A1/RConn1 -- Ideal Switch1/LConn1

== system HEV_Electrical_Lib/Mean Value/Synchronous Motor & Drive/Three-phase Inverter/Id computation ==
  m : Inport
  Vdc : Inport  Port=2
  Demux : Subsystem
  Demux1 : Subsystem
  Gain : Gain  Gain=Ron
  Math Function : Math  Operator=magnitude^2  SignedPower=on
  Math Function1 : Math  Operator=magnitude^2  SignedPower=on
  Math Function2 : Math  Operator=magnitude^2  SignedPower=on
  Product1 : Product  Inputs=*/  SaturateOnIntegerOverflow=on  OutDataTypeStr=Inherit: Same as first input
  Sum1 : Sum  Inputs=+++  SaturateOnIntegerOverflow=on
  Sum2 : Sum  Inputs=|++  SaturateOnIntegerOverflow=on
  Sum3 : Sum  SaturateOnIntegerOverflow=on
  Unit Delay1 : UnitDelay  SampleTime=Ts  HasFrameUpgradeWarning=on
  Unit Delay4 : UnitDelay  InitialCondition=1  SampleTime=Ts  HasFrameUpgradeWarning=on
  Vac x Ia : Product  SaturateOnIntegerOverflow=on  OutDataTypeStr=Inherit: Same as first input
  Vbc x Ib : Product  SaturateOnIntegerOverflow=on  OutDataTypeStr=Inherit: Same as first input
  Zero avoider : Saturate  UpperLimit=inf  LowerLimit=1
  Id : Outport  VectorParamsAs1DForOutWhenUnconnected=off
  wires:
  Zero avoider/1 -> Product1/2
  Product1/1 -> Id/1
  Gain/1 -> Sum2/2
  Demux/3(Vbc) -> Vbc x Ib/1
  Demux/4(Ib) -> Vbc x Ib/2
  Demux/2(Ia) -> Vac x Ia/2
  Demux/1(Vac) -> Vac x Ia/1
  Vdc/1 -> Unit Delay4/1
  Vbc x Ib/1 -> Sum3/2
  Vac x Ia/1 -> Sum3/1
  m/1 -> Demux/1(m), Demux1/1(m)
  Unit Delay1/1 -> Product1/1
  Unit Delay4/1 -> Zero avoider/1
  Demux1/1(Ia) -> Math Function/1
  Demux1/2(Ib) -> Math Function1/1
  Demux1/3(Ic) -> Math Function2/1
  Math Function1/1 -> Sum1/2
  Math Function/1 -> Sum1/1
  Math Function2/1 -> Sum1/3
  Sum1/1 -> Gain/1
  Sum3/1 -> Sum2/1
  Sum2/1 -> Unit Delay1/1

== system HEV_Electrical_Lib/Mean Value/Synchronous Motor & Drive/Three-phase Inverter/Limit detection ==
  note: Low pass filter
  note: Low pass filter
  note: Limit = 1 saturation mode (voltage mode)
      | Limit = 0 normal mode (current mode)
  Vcc : Inport
  ctrl : Inport  Port=2
  Bus Selector1 : BusSelector  OutputSignals=m.Stator current is_d (A),m.Stator current is_q (A),m.Rotor speed wm (rad/s)  OutputAsBus=on
  Discrete Transfer Fcn1 : DiscreteTransferFcn  Numerator=[1-exp(-Ts*Fcs*2*pi)]  Denominator=[1 -exp(-Ts*Fcs*2*pi)]  SampleTime=Ts
  Discrete Transfer Fcn3 : DiscreteTransferFcn  Numerator=[1-exp(-Ts*Fcs*2*pi)]  Denominator=[1 -exp(-Ts*Fcs*2*pi)]  SampleTime=Ts
  Gain1 : Gain  Gain=0.9  SaturateOnIntegerOverflow=on  OutDataTypeStr=Inherit: Same as input  ParamDataTypeStr=Inherit: Same as input
  "Internal Vcc " : Fcn  Expr=pi/2*sqrt((Resistance*u(1)-Lq*p*u(3)*u(2))^2+(Resistance*u(2)+Ld*p*u(3)*u(1)+Flux*p*u(3))^2)
  Relational Operator : RelationalOperator  Operator=>  OutDataTypeStr=boolean  InputSameDT=off
  Relational Operator2 : RelationalOperator  Operator=<  OutDataTypeStr=boolean  InputSameDT=off
  S-R Flip-Flop : simulink_extras/Flip Flops/S-R Flip-Flop  initial_condition=0
  Terminator : Terminator
  Limit : Outport  VectorParamsAs1DForOutWhenUnconnected=off
  wires:
  S-R Flip-Flop/2 -> Terminator/1
  Discrete Transfer Fcn3/1 -> Relational Operator/2, Gain1/1
  Gain1/1 -> Relational Operator2/2
  Discrete Transfer Fcn1/1 -> Relational Operator2/1, Relational Operator/1
  "Internal Vcc "/1 -> Discrete Transfer Fcn1/1
  Bus Selector1/1 -> "Internal Vcc "/1
  ctrl/1 -> Bus Selector1/1
  S-R Flip-Flop/1 -> Limit/1
  Relational Operator2/1 -> S-R Flip-Flop/2
  Relational Operator/1 -> S-R Flip-Flop/1
  Vcc/1 -> Discrete Transfer Fcn3/1

== system HEV_Electrical_Lib/Mean Value/Synchronous Motor & Drive/Three-phase Inverter/Output Resistance correction ==
  note: Vabc
  ctrl : Inport
  1/R : Gain  Gain=1/(100*Resistance)  SaturateOnIntegerOverflow=on  OutDataTypeStr=Inherit: Same as input  ParamDataTypeStr=Inherit: Same as input
  Bus Selector1 : BusSelector  OutputSignals=m.Stator voltage Vs_d (V),m.Stator voltage Vs_q (V),m.Rotor angle thetam (rad)
  Constant : Constant  Value=0
  Discrete Transfer Fcn1 : DiscreteTransferFcn  Numerator=[1-exp(-Ts/.001)]  Denominator=[1 -exp(-Ts/.001)]  SampleTime=Ts
  Discrete Transfer Fcn2 : DiscreteTransferFcn  Numerator=[1-exp(-Ts/.001)]  Denominator=[1 -exp(-Ts/.001)]  SampleTime=Ts
  Fcn : Fcn  Expr=sin(u)
  Fcn1 : Fcn  Expr=cos(u)
  Mux4 : Mux  Inputs=3
  Mux5 : Mux  Inputs=2
  dq0_to_abc Transformation : powerlib_extras/Measurements/dq0_to_abc Transformation
  poles : Gain  Gain=p  SaturateOnIntegerOverflow=on  OutDataTypeStr=Inherit: Same as input  ParamDataTypeStr=Inherit: Same as input
  "Iabc_r " : Outport  VectorParamsAs1DForOutWhenUnconnected=off
  wires:
  poles/1 -> Fcn/1, Fcn1/1
  Bus Selector1/3 -> poles/1  "<Rotor angle thetam (rad)>"
  Discrete Transfer Fcn1/1 -> Mux4/1
  Discrete Transfer Fcn2/1 -> Mux4/2
  dq0_to_abc Transformation/1 -> 1/R/1
  Constant/1 -> Mux4/3
  Mux5/1 -> dq0_to_abc Transformation/2
  Fcn1/1 -> Mux5/2
  Fcn/1 -> Mux5/1
  Mux4/1 -> dq0_to_abc Transformation/1
  ctrl/1 -> Bus Selector1/1
  Bus Selector1/1 -> Discrete Transfer Fcn1/1  "<Stator voltage Vs_d (V)>"
  Bus Selector1/2 -> Discrete Transfer Fcn2/1  "<Stator voltage Vs_q (V)>"
  1/R/1 -> "Iabc_r "/1

== system HEV_Electrical_Lib/Mean Value/Synchronous Motor & Drive/VECT controller/Current Regulator ==
  Iabc* : Inport
  Iabc : Inport  Port=2
  Demux1 : Demux  Outputs=3
      settings: DisplayOption=none
  Demux2 : Demux  Outputs=3
      settings: DisplayOption=none
  Mux1 : Mux  Inputs=2
  Relay : Relay  OnSwitchValue=0  OffSwitchValue=0
  Relay1 : Relay  OnSwitchValue=0  OffSwitchValue=0
  Relay2 : Relay  OnSwitchValue=0  OffSwitchValue=0
  Sum : Sum  Inputs=-+  InputSameDT=on  SaturateOnIntegerOverflow=on  OutDataTypeStr=Inherit: Same as first input
  Sum1 : Sum  Inputs=-+  InputSameDT=on  SaturateOnIntegerOverflow=on  OutDataTypeStr=Inherit: Same as first input
  Sum2 : Sum  Inputs=-+  InputSameDT=on  SaturateOnIntegerOverflow=on  OutDataTypeStr=Inherit: Same as first input
  Sum3 : Sum  Inputs=+-
  Sum4 : Sum  Inputs=+-
  Pulses : Outport  InitialOutput=0  VectorParamsAs1DForOutWhenUnconnected=off
  wires:
  Sum4/1 -> Mux1/2
  Sum3/1 -> Mux1/1
  Relay2/1 -> Sum4/2
  Relay1/1 -> Sum4/1, Sum3/2
  Relay/1 -> Sum3/1
  Iabc*/1 -> Demux2/1
  Demux2/1 -> Sum/2
  Demux2/2 -> Sum1/2
  Demux2/3 -> Sum2/2
  Demux1/3 -> Sum2/1
  Sum2/1 -> Relay2/1
  Iabc/1 -> Demux1/1
  Mux1/1 -> Pulses/1
  Demux1/2 -> Sum1/1
  Demux1/1 -> Sum/1
  Sum1/1 -> Relay1/1
  Sum/1 -> Relay/1

== system HEV_Electrical_Lib/Mean Value/Synchronous Motor & Drive/VECT controller/DQ-ABC ==
  "Iq* " : Inport
  "Id* " : Inport  Port=2
  Teta : Inport  Port=3
  Fcn : Fcn  Expr=sin(u)
  Fcn1 : Fcn  Expr=cos(u)
  Gain2 : Gain  SaturateOnIntegerOverflow=on  OutDataTypeStr=Inherit: Same as input  ParamDataTypeStr=Inherit: Same as input
  Gain3 : Gain  SaturateOnIntegerOverflow=on  OutDataTypeStr=Inherit: Same as input  ParamDataTypeStr=Inherit: Same as input
  Gain4 : Gain  SaturateOnIntegerOverflow=on  OutDataTypeStr=Inherit: Same as input  ParamDataTypeStr=Inherit: Same as input
  Mux : Mux
  Mux2 : Mux  Inputs=3
  ia : Fcn  Expr=-u[3]*u[2] + u[4]*u[1]
  ib : Fcn  Expr=(-u[1]+1.7320508*u[2])*u[4]*0.5+(u[2]+1.7320508*u[1])*u[3]*0.5
  ic : Sum  Inputs=--  InputSameDT=on  SaturateOnIntegerOverflow=on  OutDataTypeStr=Inherit: Same as first input
  Iabc* : Outport  InitialOutput=0  VectorParamsAs1DForOutWhenUnconnected=off
  wires:
  ib/1 -> ic/1, Gain3/1
  ia/1 -> ic/2, Gain2/1
  Gain2/1 -> Mux2/1
  Gain4/1 -> Mux2/3
  ic/1 -> Gain4/1
  Gain3/1 -> Mux2/2
  "Iq* "/1 -> Mux/4
  "Id* "/1 -> Mux/3
  Teta/1 -> Fcn/1, Fcn1/1
  Mux/1 -> ia/1, ib/1
  Mux2/1 -> Iabc*/1
  Fcn1/1 -> Mux/1
  Fcn/1 -> Mux/2

== system HEV_Electrical_Lib/Mean Value/Synchronous Motor & Drive/VECT controller/Zero crossing detector ==
  En : Inport
  Iabc* : Inport  Port=2
  D Latch : simulink_extras/Flip Flops/D Latch
  D Latch1 : simulink_extras/Flip Flops/D Latch
  D Latch2 : simulink_extras/Flip Flops/D Latch
  Data Type Conversion : DataTypeConversion  SaturateOnIntegerOverflow=off  RndMeth=Floor
  Data Type Conversion2 : DataTypeConversion  SaturateOnIntegerOverflow=off  RndMeth=Floor
  Demux : Demux  Outputs=3
  Hit Crossing : HitCross
  Mux : Mux  Inputs=3
  Terminator : Terminator
  Terminator1 : Terminator
  Terminator2 : Terminator
  Enable : Outport  VectorParamsAs1DForOutWhenUnconnected=off
  wires:
  D Latch2/2 -> Terminator2/1
  D Latch1/2 -> Terminator1/1
  D Latch/2 -> Terminator/1
  Data Type Conversion2/1 -> Enable/1
  Iabc*/1 -> Hit Crossing/1
  En/1 -> Data Type Conversion/1
  Demux/1 -> D Latch/2
  Mux/1 -> Data Type Conversion2/1
  D Latch2/1 -> Mux/3
  D Latch1/1 -> Mux/2
  D Latch/1 -> Mux/1
  Demux/3 -> D Latch2/2
  Demux/2 -> D Latch1/2
  Hit Crossing/1 -> Demux/1
  Data Type Conversion/1 -> D Latch2/1, D Latch1/1, D Latch/1

== system HEV_Electrical_Lib/Subsystem/System Level/DC-DC Converter/Calcuate Input Current Pout+PLoss = Pin ==
  note: Power Output
  note: Total Power
  Input^2 : fl_lib/Physical Signals/Functions/PS Math Function  fcn_choice=7  v=1
  No Div By 0 : fl_lib/Physical Signals/Nonlinear Operators/PS Max
      settings: InternalSimscapePortConfiguration="{\"Bottom\":[],\"Left\":[{\"id\":\"I1\",\"label\":\"\",\"type\":\"input\"},{\"id\":\"I2\",\"label\":\"\",\"type\":\"input\"}],\"Right\":[{\"id\":\"O\",\"label\":\"\",\"type\":\"output\"}],\"Top\":[]}"
  PS Add : fl_lib/Physical Signals/Functions/PS Add
  PS Constant : fl_lib/Physical Signals/Sources/PS Constant  constant=HEV_Param.DCDCConv.MinVin V
  PS Divide : fl_lib/Physical Signals/Functions/PS Divide
  PS Product : fl_lib/Physical Signals/Functions/PS Product
  RLoadLoss : fl_lib/Physical Signals/Functions/PS Gain  gain=RLoadLoss Ohm
  V_In : PMIOPort  Side=Left
  Iout : PMIOPort  Port=2  Side=Left
  Vout : PMIOPort  Port=3  Side=Left
  I_Input : PMIOPort  Port=4  Side=Right
  P Loss : PMIOPort  Port=5  Side=Right
  connections:
  I_Input/RConn1 -- PS Divide/RConn1
  Vout/RConn1 -- PS Product/LConn2
  Input^2/LConn1 -- PS Product/LConn1 -- Iout/RConn1
  RLoadLoss/LConn1 -- Input^2/RConn1
  PS Add/LConn2 -- PS Product/RConn1
  PS Add/LConn1 -- RLoadLoss/RConn1 -- P Loss/RConn1
  No Div By 0/LConn1 -- PS Constant/RConn1
  V_In/RConn1 -- No Div By 0/LConn2
  No Div By 0/RConn1 -- PS Divide/LConn2
  PS Add/RConn1 -- PS Divide/LConn1

== system HEV_Electrical_Lib/Subsystem/System Level/DC-DC Converter/Control Bus Voltage ==
  Ki : fl_lib/Physical Signals/Functions/PS Gain  gain=Ki 1/s
  Kp : fl_lib/Physical Signals/Functions/PS Gain  gain=Kp
  PS Add1 : fl_lib/Physical Signals/Functions/PS Add
  PS Integrator : fl_lib/Physical Signals/Linear Operators/PS Integrator  reset_method=foundation.enum.IntegratorResetSpec.None  initial_condition_spec=foundation.enum.IntegratorICSpec.Internal  saturation_spec=foundation.enum.IntegratorSaturationSpec.None  saturation_source_spec=foundation.enum.IntegratorSaturationSourceSpec.Internal  x0=Vout V  xu=inf s  xl=-inf s
  PS Subtract : fl_lib/Physical Signals/Functions/PS Subtract
  Vmeas : PMIOPort  Side=Left
  Vref : PMIOPort  Port=2  Side=Left
  VBus : PMIOPort  Port=3  Side=Right
  connections:
  PS Integrator/RConn1 -- PS Add1/LConn1
  VBus/RConn1 -- PS Add1/RConn1
  Vref/RConn1 -- PS Subtract/LConn1
  Vmeas/RConn1 -- PS Subtract/LConn2
  PS Integrator/LConn1 -- Ki/RConn1
  Ki/LConn1 -- PS Subtract/RConn1 -- Kp/LConn1
  PS Add1/LConn2 -- Kp/RConn1

== system HEV_Electrical_Lib/Subsystem/System Level/DC-DC Converter/Current Sensor ==
  Current Sensor : fl_lib/Electrical/Electrical Sensors/Current Sensor
  PS-Simulink Converter : nesl_utility/PS-Simulink Converter  PhysicalDomain=network_engine_domain  SubClassName=ps_output  LeftPortType=input  RightPortType=output  PseudoPeriodic=off  Frequencies=[]  VectorFormat=1-D array  Unit=1  AffineConversion=off
  I : PMIOPort  Side=Right
  + : PMIOPort  Port=2  Side=Left
  - : PMIOPort  Port=3  Side=Right
  tag scope: I_out=global
  wires:
  PS-Simulink Converter/1 -> [I_out]
  connections:
  Current Sensor/RConn1 -- I/RConn1 -- PS-Simulink Converter/LConn1
  +/RConn1 -- Current Sensor/LConn1
  -/RConn1 -- Current Sensor/RConn2

== system HEV_Electrical_Lib/Subsystem/System Level/DC-DC Converter/Subsystem3 ==
  PS-Simulink Converter : nesl_utility/PS-Simulink Converter  PhysicalDomain=network_engine_domain  SubClassName=ps_output  LeftPortType=input  RightPortType=output  PseudoPeriodic=off  Frequencies=[]  VectorFormat=1-D array  Unit=A  AffineConversion=off
  Out : PMIOPort  Tag=PMCPort  Side=Right
  In : PMIOPort  Tag=PMCPort  Port=2  Side=Left
  tag scope: I_in=global
  wires:
  PS-Simulink Converter/1 -> [I_in]
  connections:
  PS-Simulink Converter/LConn1 -- Out/RConn1 -- In/RConn1
